simulink model "motor_model_final"  (R2020a)
settings: Solver=VariableStepAuto  StartTime=0.0  StopTime=20  RelTol=1e-3
undefined symbols (not defined in the file or in its folder): ctrl_deadZone, k_motor, Km, L, Motor, Motor_Lib, R, sigbuilder_block, X, Y, Z
libraries: fl_lib x45, nesl_utility x36, ee_lib x9, sm_lib x8, sdl_lib x3, simulink x1
(part 1 of 2)
settings Model: Creator=RAJENDRA PHUTANE  LastModifiedBy=RAJENDRA PHUTANE

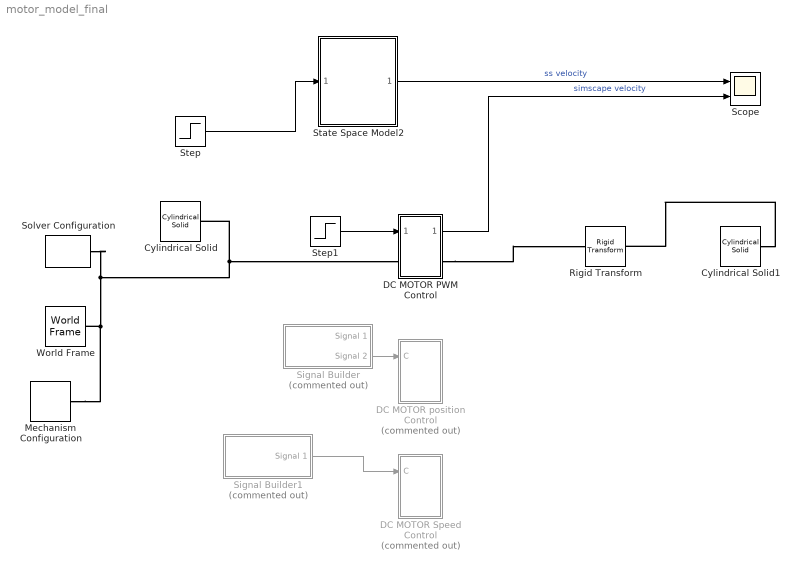
== system motor_model_final ==
  Cylindrical Solid : sm_lib/Body Elements/Cylindrical Solid  GraphicAmbientColor=[0.15 0.15 0.15 1.0]  BasedOnType=Density  CenterOfMass=[0 0 0]  CenterOfMassUnits=m  GraphicDiffuseColor=[0.5 0.5 0.5]  CylinderLength=1  CylinderLengthUnits=m  CylinderRadius=0.007  CylinderRadiusUnits=m  Density=1000  DensityUnits=kg/m^3  DoExposeReferenceFrame=on  GraphicEmissiveColor=[0.0 0.0 0.0 1.0]  ExportEntireGeometry=off  SerializedFrames=<Frames/>  MarkerShape=Sphere  MarkerSize=10  GraphicType=FromGeometry  InertiaType=CalculateFromGeometry  Mass=1  MassUnits=kg  MomentsOfInertia=[1 1 1]  MomentsOfInertiaUnits=kg*m^2  GraphicOpacity=1.0  ProductsOfInertia=[0 0 0]  ProductsOfInertiaUnits=kg*m^2  GraphicShininess=75  GraphicSpecularColor=[0.5 0.5 0.5 1.0]  GraphicVisPropType=SimpleVisualProperties
  Cylindrical Solid1 : sm_lib/Body Elements/Cylindrical Solid  GraphicAmbientColor=[0.15 0.15 0.15 1.0]  BasedOnType=Mass  CenterOfMass=[0 0 0]  CenterOfMassUnits=m  GraphicDiffuseColor=[0.5 0.5 0.5]  CylinderLength=0.01  CylinderLengthUnits=m  CylinderRadius=0.017  CylinderRadiusUnits=m  Density=1000  DensityUnits=kg/m^3  DoExposeReferenceFrame=on  GraphicEmissiveColor=[0.0 0.0 0.0 1.0]  ExportEntireGeometry=off  SerializedFrames=<Frames/>  MarkerShape=Sphere  MarkerSize=10  GraphicType=FromGeometry  InertiaType=CalculateFromGeometry  Mass=19.4  MassUnits=g  MomentsOfInertia=[1 1 1]  MomentsOfInertiaUnits=kg*m^2  GraphicOpacity=1.0  ProductsOfInertia=[0 0 0]  ProductsOfInertiaUnits=kg*m^2  GraphicShininess=75  GraphicSpecularColor=[0.5 0.5 0.5 1.0]  GraphicVisPropType=SimpleVisualProperties
  DC MOTOR PWM Control : Subsystem
  DC MOTOR Speed Control : Subsystem  Commented=on
  DC MOTOR position Control : Subsystem  Commented=on
  Mechanism Configuration : sm_lib/Utilities/Mechanism Configuration  UniformGravity=Constant  GravityVector=[0 0 -9.80665]  GravityUnits=m/s^2  LinearizationDelta=0.001
  Rigid Transform : sm_lib/Frames and Transforms/Rigid Transform  TranslationMethod=StandardAxis  TranslationStandardOffset=0.5  TranslationLengthUnit=m  TranslationStandardAxis=+Z  TranslationCartesianOffset=[0 0 0]  TranslationROffset=0  TranslationROffsetUnits=m  TranslationZOffset=0  TranslationZOffsetUnits=m  TranslationThetaOffset=0  TranslationThetaOffsetUnits=deg  RotationMethod=None  RotationAngleUnits=deg  RotationStandardAxis=+Z  RotationAngle=0.0  RotationArbitraryAxis=[0 0 1]  FollAlignAxisA=+X  BaseAlignAxisA=+Y  FollAlignAxisB=+Y  BaseAlignAxisB=+Z  RotationSequenceAxes=FollowerAxes  RotationSequence=XYX  RotationSequenceAngles=[0 0 0]  RotationSequenceAnglesUnits=deg  RotationMatrix=[1 0 0; 0 1 0; 0 0 1]
  Scope : Scope  NumInputPorts=2
  Signal Builder : Subsystem  Tag=STV Subsys  Commented=on  LoadFcn=sigbuilder_block('load');  StartFcn=sigbuilder_block('start');  StopFcn=sigbuilder_block('stop');  ClipboardFcn=sigbuilder_block('clipboard');  mask(Sigbuilder block){tuvar=[0:10]}
      mask help: Simulink:masks:SigbuilderBlock_MD
      mask init:
      | if ~strcmp(get_param(bdroot(gcbh),'SimulationStatus'),'stopped') tuvar = sigbuilder_block('maskInit'); end
      settings: CopyFcn=sigbuilder_block('copy');  DeleteFcn=sigbuilder_block('delete');  ModelCloseFcn=sigbuilder_block('modelClose');  PreSaveFcn=sigbuilder_block('preSave');  PauseFcn=sigbuilder_block('pause');  ContinueFcn=sigbuilder_block('continue');  NameChangeFcn=sigbuilder_block('namechange');  OpenFcn=sigbuilder_block('open',[437.6 199.2 550.4 400 ]);  CloseFcn=sigbuilder_block('close');
      mask Display: plot(0, 0, 100, 100,[2, 2, 32, 32, 2], [68, 8, 8, 68, 68],[32, 2], [38, 38], [32, 19, 2],[53, 60, 44], [32, 17, 17, 2],[16, 16, 31, 31]);txt = getActiveGroup(gcbh);text(2, 100, txt,'verticalAlignment', 'top');
  Signal Builder1 : Subsystem  Tag=STV Subsys  Commented=on  LoadFcn=sigbuilder_block('load');  StartFcn=sigbuilder_block('start');  StopFcn=sigbuilder_block('stop');  ClipboardFcn=sigbuilder_block('clipboard');  mask(Sigbuilder block){tuvar=[0:10]}
      mask help: Simulink:masks:SigbuilderBlock_MD
      mask init:
      | if ~strcmp(get_param(bdroot(gcbh),'SimulationStatus'),'stopped') tuvar = sigbuilder_block('maskInit'); end
      settings: CopyFcn=sigbuilder_block('copy');  DeleteFcn=sigbuilder_block('delete');  ModelCloseFcn=sigbuilder_block('modelClose');  PreSaveFcn=sigbuilder_block('preSave');  PauseFcn=sigbuilder_block('pause');  ContinueFcn=sigbuilder_block('continue');  NameChangeFcn=sigbuilder_block('namechange');  OpenFcn=sigbuilder_block('open',[437.6 199.2 550.4 400 ]);  CloseFcn=sigbuilder_block('close');
      mask Display: plot(0, 0, 100, 100,[2, 2, 32, 32, 2], [68, 8, 8, 68, 68],[32, 2], [38, 38], [32, 19, 2],[53, 60, 44], [32, 17, 17, 2],[16, 16, 31, 31]);txt = getActiveGroup(gcbh);text(2, 100, txt,'verticalAlignment', 'top');
  Solver Configuration : nesl_utility/Solver Configuration  PhysicalDomain=network_engine_domain  SubClassName=solver  LeftPortType=input  RightPortType=generic  Tones=[]  Harmonics=[]  SimulateNoise=off  Profile=off  UseLocalSampling=off  EnableSwitchedLinearOptims=on  FrequencyDomain=off  UseCCode=off  RelTol=0.001  AbsTol=1e-06  MinStep=1e-09  ToWorkspace=off  RevertToSquareIcSolve=off  NumHomotopyIterations=100  PhasorMode=off  PhasorModeNumHarmonics=1  DoDC=off  ResidualTolerance=1e-09  UseLocalSolver=off  LocalSolverChoice=NE_BACKWARD_EULER_ADVANCER  LocalSolverSampleTime=0.001  DoFixedCost=off  MaxNonlinIter=3  MaxModeIter=2  LinearAlgebra=auto  EquationFormulation=NE_TIME_EF  DelaysMemoryBudget=1024  AutomaticFiltering=on  FilteringTimeConstant=0.001  PartitionStorageMethod=AS_NEEDED  PartitionMemoryBudget=1024  PartitionMethod=ROBUST
  State Space Model2 : Subsystem  AncestorBlock=DCMotorLibrary/State Space Model  mask(DC Motor){K=Km, R=R, L=L, b=0.0005625, J=0.0001}
      mask prompts: K "Torque Constant:"; R "Armature Resistance:"; L "Armature Inductance:"; b "Damping Coefficient:"; J "Rotor Inertia:"
      mask help:
      | This block simulates a basic brushed DC Motor with voltage input and rotor
      | angle in degrees as the output.
      mask Display: image(imread('dcmotor.jpg'))
  Step : Step  Time=5  Before=-12  After=12  SampleTime=0
  Step1 : Step  Time=5  Before=-255  After=255  SampleTime=0
  World Frame : sm_lib/Frames and Transforms/World Frame
  wires:
  Step1/1 -> DC MOTOR PWM Control/1(PWM)
  Signal Builder/2(Signal 2) -> DC MOTOR position Control/1(C)
  Signal Builder1/1(Signal 1) -> DC MOTOR Speed Control/1(C)
  DC MOTOR PWM Control/1(Outport) -> Scope/2  "simscape velocity"
  Step/1 -> State Space Model2/1(Voltage)
  State Space Model2/1(Velocity) -> Scope/1  "ss velocity"
  connections:
  Cylindrical Solid1/RConn1 -- Rigid Transform/RConn1
  Mechanism Configuration/RConn1 -- Solver Configuration/RConn1 -- DC MOTOR PWM Control/LConn1 -- Cylindrical Solid/RConn1 -- World Frame/RConn1
  DC MOTOR PWM Control/RConn1 -- Rigid Transform/LConn1

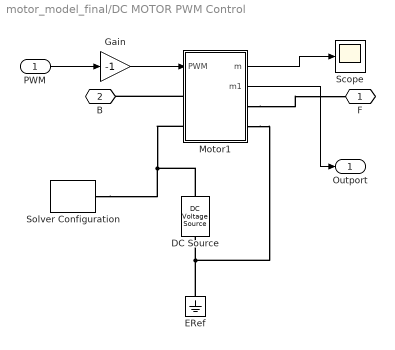
== system motor_model_final/DC MOTOR PWM Control ==
  PWM : Inport
  DC Source : fl_lib/Electrical/Electrical Sources/DC Voltage Source  v0=12 V
  ERef : fl_lib/Electrical/Electrical Elements/Electrical Reference
  Gain : Gain  Gain=-1
  Motor1 : Subsystem  VariantControl=Motor
      mask Display: image('youBot_Arm_Actuation_Motor_Motor_IMAGE.jpg');
  Scope : Scope
  Solver Configuration : nesl_utility/Solver Configuration  PhysicalDomain=network_engine_domain  SubClassName=solver  LeftPortType=input  RightPortType=generic  Tones=[]  Harmonics=[]  SimulateNoise=off  Profile=off  UseLocalSampling=off  EnableSwitchedLinearOptims=on  FrequencyDomain=off  UseCCode=off  RelTol=0.001  AbsTol=1e-06  MinStep=1e-09  ToWorkspace=off  RevertToSquareIcSolve=off  NumHomotopyIterations=100  PhasorMode=off  PhasorModeNumHarmonics=1  DoDC=off  ResidualTolerance=1e-09  UseLocalSolver=off  LocalSolverChoice=NE_BACKWARD_EULER_ADVANCER  LocalSolverSampleTime=0.001  DoFixedCost=off  MaxNonlinIter=3  MaxModeIter=2  LinearAlgebra=auto  EquationFormulation=NE_TIME_EF  DelaysMemoryBudget=1024  AutomaticFiltering=on  FilteringTimeConstant=0.001  PartitionStorageMethod=AS_NEEDED  PartitionMemoryBudget=1024  PartitionMethod=ROBUST
  F : PMIOPort  Side=Right
  B : PMIOPort  Port=2  Side=Left
  Outport : Outport
  wires:
  PWM/1 -> Gain/1
  Motor1/1(m) -> Scope/1
  Gain/1 -> Motor1/1(PWM)
  Motor1/2(m1) -> Outport/1
  connections:
  Motor1/RConn1 -- F/RConn1
  Motor1/LConn1 -- B/RConn1
  Solver Configuration/RConn1 -- Motor1/LConn2 -- DC Source/LConn1
  ERef/LConn1 -- Motor1/RConn2 -- DC Source/RConn1

== system motor_model_final/DC MOTOR Speed Control ==
  C : Inport
  DC Source : fl_lib/Electrical/Electrical Sources/DC Voltage Source  v0=12 V
  ERef : fl_lib/Electrical/Electrical Elements/Electrical Reference
  Motor1 : Subsystem  VariantControl=Motor
      mask Display: image('youBot_Arm_Actuation_Motor_Motor_IMAGE.jpg');
  Solver Configuration : nesl_utility/Solver Configuration  PhysicalDomain=network_engine_domain  SubClassName=solver  LeftPortType=input  RightPortType=generic  Tones=[]  Harmonics=[]  SimulateNoise=off  Profile=off  UseLocalSampling=off  EnableSwitchedLinearOptims=on  FrequencyDomain=off  UseCCode=off  RelTol=0.001  AbsTol=1e-06  MinStep=1e-09  ToWorkspace=off  RevertToSquareIcSolve=off  NumHomotopyIterations=100  PhasorMode=off  PhasorModeNumHarmonics=1  DoDC=off  ResidualTolerance=1e-09  UseLocalSolver=off  LocalSolverChoice=NE_BACKWARD_EULER_ADVANCER  LocalSolverSampleTime=0.001  DoFixedCost=off  MaxNonlinIter=3  MaxModeIter=2  LinearAlgebra=auto  EquationFormulation=NE_TIME_EF  DelaysMemoryBudget=1024  AutomaticFiltering=on  FilteringTimeConstant=0.001  PartitionStorageMethod=AS_NEEDED  PartitionMemoryBudget=1024  PartitionMethod=ROBUST
  Terminator : Terminator
  F : PMIOPort  Side=Right
  B : PMIOPort  Port=2  Side=Left
  wires:
  C/1 -> Motor1/1(C)
  Motor1/1(m) -> Terminator/1
  connections:
  Motor1/RConn1 -- F/RConn1
  Motor1/LConn1 -- B/RConn1
  Solver Configuration/RConn1 -- Motor1/LConn2 -- DC Source/LConn1
  ERef/LConn1 -- Motor1/RConn2 -- DC Source/RConn1

== system motor_model_final/DC MOTOR position Control ==
  C : Inport
  DC Source : fl_lib/Electrical/Electrical Sources/DC Voltage Source  v0=12 V
  ERef : fl_lib/Electrical/Electrical Elements/Electrical Reference
  Motor1 : Subsystem  VariantControl=Motor
      mask Display: image('youBot_Arm_Actuation_Motor_Motor_IMAGE.jpg');
  Solver Configuration : nesl_utility/Solver Configuration  PhysicalDomain=network_engine_domain  SubClassName=solver  LeftPortType=input  RightPortType=generic  Tones=[]  Harmonics=[]  SimulateNoise=off  Profile=off  UseLocalSampling=off  EnableSwitchedLinearOptims=on  FrequencyDomain=off  UseCCode=off  RelTol=0.001  AbsTol=1e-06  MinStep=1e-09  ToWorkspace=off  RevertToSquareIcSolve=off  NumHomotopyIterations=100  PhasorMode=off  PhasorModeNumHarmonics=1  DoDC=off  ResidualTolerance=1e-09  UseLocalSolver=off  LocalSolverChoice=NE_BACKWARD_EULER_ADVANCER  LocalSolverSampleTime=0.001  DoFixedCost=off  MaxNonlinIter=3  MaxModeIter=2  LinearAlgebra=auto  EquationFormulation=NE_TIME_EF  DelaysMemoryBudget=1024  AutomaticFiltering=on  FilteringTimeConstant=0.001  PartitionStorageMethod=AS_NEEDED  PartitionMemoryBudget=1024  PartitionMethod=ROBUST
  Terminator : Terminator
  F : PMIOPort  Side=Right
  B : PMIOPort  Port=2  Side=Left
  wires:
  Motor1/1(m) -> Terminator/1
  C/1 -> Motor1/1(C)
  connections:
  DC Source/RConn1 -- Motor1/RConn2 -- ERef/LConn1
  DC Source/LConn1 -- Motor1/LConn2 -- Solver Configuration/RConn1
  Motor1/LConn1 -- B/RConn1
  Motor1/RConn1 -- F/RConn1

== system motor_model_final/Signal Builder ==
  Demux : Demux  Tag=STV Demux  Outputs=2
      settings: DisplayOption=none
  FromWs : FromWorkspace  Tag=STV FromWs  VariableName=tuvar
      SigBuilderData=|
      | common.afterFinalStr = 'Extrapolate'
      | common.sampleTime = 0
      | dataSet.timeRange = [0 10]
      | dataSet.name = 'Group 1'
      | sbobj.Groups.Name = 'Group 1'
      | sbobj.Groups.Signals(1).Name = 'Signal 1'
      | sbobj.Groups.Signals(1).XData = [0 4 4 6 6 10]
      | sbobj.Groups.Signals(1).YData = [0 0 1 1 0 0]
      | sbobj.Groups.Signals(2).Name = 'Signal 2'
      | sbobj.Groups.Signals(2).XData = [0 2 3 4 5 6 10]
      | sbobj.Groups.Signals(2).YData = [0 180 180 90 90 -90 -90]
  Signal 1 : Outport  Tag=STV Outport
  Signal 2 : Outport  Tag=STV Outport  Port=2
  wires:
  Demux/1 -> Signal 1/1
  FromWs/1 -> Demux/1
  Demux/2 -> Signal 2/1

== system motor_model_final/Signal Builder1 ==
  Demux : Demux  Tag=STV Demux  Outputs=1
      settings: DisplayOption=none
  FromWs : FromWorkspace  Tag=STV FromWs  VariableName=tuvar
      SigBuilderData=|
      | common.afterFinalStr = 'Extrapolate'
      | common.sampleTime = 0
      | dataSet.timeRange = [0 20]
      | dataSet.name = 'Group 1'
      | sbobj.Groups.Name = 'Group 1'
      | sbobj.Groups.Signals.Name = 'Signal 1'
      | sbobj.Groups.Signals.XData = [0 1 1 3.98 3.98 6 6 9 9 14 14 20]
      | sbobj.Groups.Signals.YData = [0 0 0.6 0.6 0 0 -0.5 -0.5 0 0.5 -0.685 -0.685]
      | sbobj.Groups.TimeRange = [0 20]
  Signal 1 : Outport  Tag=STV Outport
  wires:
  Demux/1 -> Signal 1/1
  FromWs/1 -> Demux/1

== system motor_model_final/State Space Model2 ==
  Voltage : Inport
  State-Space : StateSpace  A=[-b/J K/J; -K/L -R/L]  B=[0; 1/L]  C=[1 0]  D=[0]  InitialCondition=0
  Velocity : Outport
  wires:
  Voltage/1 -> State-Space/1
  State-Space/1 -> Velocity/1

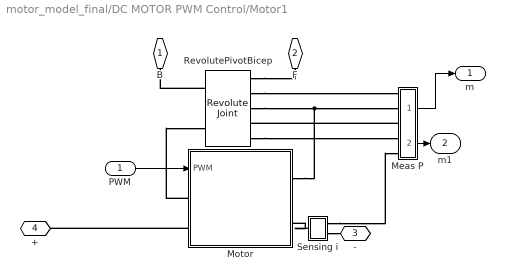
== system motor_model_final/DC MOTOR PWM Control/Motor1 ==
  PWM : Inport
  Meas P : Subsystem  Tag=CustomStyle
      mask Display: disp('m')
  Motor : Subsystem  AncestorBlock=Motor_Lib/Motor  VariantControl=Motor
  RevolutePivotBicep : sm_lib/Joints/Revolute Joint  JointMode=Normal  SenseConstraintForce=on  SenseConstraintForceX=off  SenseConstraintForceY=off  SenseConstraintForceZ=off  SenseConstraintTorque=off  SenseConstraintTorqueX=off  SenseConstraintTorqueY=off  SenseConstraintTorqueZ=off  SenseTotalForce=off  SenseTotalForceX=off  SenseTotalForceY=off  SenseTotalForceZ=off  SenseTotalTorque=off  SenseTotalTorqueX=off  SenseTotalTorqueY=off  SenseTotalTorqueZ=off  CompositeWrenchDir=FollowerOnBase  CompositeWrenchFrame=BaseFrame  EquilibriumPosition=0  EquilibriumPositionUnits=rad  SpringStiffness=0  SpringStiffnessUnits=N*m/rad  DampingCoefficient=0  DampingCoefficientUnits=N*m/(rad/s)  TorqueActuationMode=InputTorque  MotionActuationMode=ComputedMotion  SensePosition=on  SenseVelocity=on  SenseAcceleration=off  SenseTorqueForce=on  SenseLowerLimitTorqueForce=off  SenseUpperLimitTorqueForce=off  LowerLimitSpecify=off  LowerLimitBound=-90  LowerLimitBoundUnits=deg  LowerLimitStiffness=1e4  LowerLimitStiffnessUnits=N*m/deg  LowerLimitDamping=10  LowerLimitDampingUnits=N*m/(deg/s)  LowerLimitTransitionRegionWidth=0.1  LowerLimitTransitionRegionWidthUnits=deg  UpperLimitSpecify=off  UpperLimitBound=90  UpperLimitBoundUnits=deg  UpperLimitStiffness=1e4  UpperLimitStiffnessUnits=N*m/deg  UpperLimitDamping=10  UpperLimitDampingUnits=N*m/(deg/s)  UpperLimitTransitionRegionWidth=0.1  UpperLimitTransitionRegionWidthUnits=deg  PositionTargetSpecify=on  PositionTargetPriority=Low  PositionTargetValue=0  PositionTargetValueUnits=deg  VelocityTargetSpecify=off  VelocityTargetPriority=High  VelocityTargetValue=0  VelocityTargetValueUnits=deg/s
  Sensing i : Subsystem
      mask Display: disp('i')
  B : PMIOPort  Side=Left
  F : PMIOPort  Port=2  Side=Right
  - : PMIOPort  Port=3  Side=Right
  + : PMIOPort  Port=4  Side=Left
  m : Outport  VectorParamsAs1DForOutWhenUnconnected=off
  m1 : Outport  Port=2  VectorParamsAs1DForOutWhenUnconnected=off
  wires:
  PWM/1 -> Motor/1(PWM)
  Meas P/1(P) -> m/1
  Meas P/2(P1) -> m1/1
  connections:
  RevolutePivotBicep/RConn5 -- Meas P/LConn4
  Sensing i/RConn1 -- Meas P/LConn5
  Sensing i/RConn2 -- -/RConn1
  Motor/LConn2 -- +/RConn1
  Sensing i/LConn1 -- Motor/RConn2
  RevolutePivotBicep/LConn1 -- B/RConn1
  RevolutePivotBicep/RConn1 -- F/RConn1
  Motor/LConn1 -- RevolutePivotBicep/LConn2
  Motor/RConn1 -- RevolutePivotBicep/RConn3 -- Meas P/LConn2
  Meas P/LConn3 -- RevolutePivotBicep/RConn4
  RevolutePivotBicep/RConn2 -- Meas P/LConn1

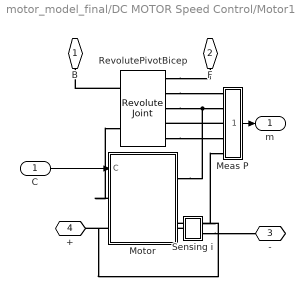
== system motor_model_final/DC MOTOR Speed Control/Motor1 ==
  C : Inport
  Meas P : Subsystem  Tag=CustomStyle
      mask Display: disp('m')
  Motor : Subsystem  AncestorBlock=Motor_Lib/Motor  VariantControl=Motor
  RevolutePivotBicep : sm_lib/Joints/Revolute Joint  JointMode=Normal  SenseConstraintForce=on  SenseConstraintForceX=off  SenseConstraintForceY=off  SenseConstraintForceZ=off  SenseConstraintTorque=off  SenseConstraintTorqueX=off  SenseConstraintTorqueY=off  SenseConstraintTorqueZ=off  SenseTotalForce=off  SenseTotalForceX=off  SenseTotalForceY=off  SenseTotalForceZ=off  SenseTotalTorque=off  SenseTotalTorqueX=off  SenseTotalTorqueY=off  SenseTotalTorqueZ=off  CompositeWrenchDir=FollowerOnBase  CompositeWrenchFrame=BaseFrame  EquilibriumPosition=0  EquilibriumPositionUnits=rad  SpringStiffness=0  SpringStiffnessUnits=N*m/rad  DampingCoefficient=0  DampingCoefficientUnits=N*m/(rad/s)  TorqueActuationMode=InputTorque  MotionActuationMode=ComputedMotion  SensePosition=on  SenseVelocity=on  SenseAcceleration=off  SenseTorqueForce=on  SenseLowerLimitTorqueForce=off  SenseUpperLimitTorqueForce=off  LowerLimitSpecify=off  LowerLimitBound=-90  LowerLimitBoundUnits=deg  LowerLimitStiffness=1e4  LowerLimitStiffnessUnits=N*m/deg  LowerLimitDamping=10  LowerLimitDampingUnits=N*m/(deg/s)  LowerLimitTransitionRegionWidth=0.1  LowerLimitTransitionRegionWidthUnits=deg  UpperLimitSpecify=off  UpperLimitBound=90  UpperLimitBoundUnits=deg  UpperLimitStiffness=1e4  UpperLimitStiffnessUnits=N*m/deg  UpperLimitDamping=10  UpperLimitDampingUnits=N*m/(deg/s)  UpperLimitTransitionRegionWidth=0.1  UpperLimitTransitionRegionWidthUnits=deg  PositionTargetSpecify=on  PositionTargetPriority=Low  PositionTargetValue=0  PositionTargetValueUnits=deg  VelocityTargetSpecify=off  VelocityTargetPriority=High  VelocityTargetValue=0  VelocityTargetValueUnits=deg/s
  Sensing i : Subsystem
      mask Display: disp('i')
  B : PMIOPort  Side=Left
  F : PMIOPort  Port=2  Side=Right
  - : PMIOPort  Port=3  Side=Right
  + : PMIOPort  Port=4  Side=Left
  m : Outport  VectorParamsAs1DForOutWhenUnconnected=off
  wires:
  C/1 -> Motor/1(C)
  Meas P/1(P) -> m/1
  connections:
  RevolutePivotBicep/RConn5 -- Meas P/LConn4
  Sensing i/RConn1 -- Meas P/LConn5
  Sensing i/RConn2 -- -/RConn1
  Motor/LConn2 -- +/RConn1
  Sensing i/LConn1 -- Motor/RConn2
  RevolutePivotBicep/LConn1 -- B/RConn1
  RevolutePivotBicep/RConn1 -- F/RConn1
  Motor/LConn1 -- RevolutePivotBicep/LConn2
  Motor/RConn1 -- Meas P/LConn2 -- RevolutePivotBicep/RConn3
  Meas P/LConn3 -- RevolutePivotBicep/RConn4
  RevolutePivotBicep/RConn2 -- Meas P/LConn1

== system motor_model_final/DC MOTOR position Control/Motor1 ==
  C : Inport
  Meas P : Subsystem  Tag=CustomStyle
      mask Display: disp('m')
  Motor : Subsystem  AncestorBlock=Motor_Lib/Motor  VariantControl=Motor
  RevolutePivotBicep : sm_lib/Joints/Revolute Joint  JointMode=Normal  SenseConstraintForce=on  SenseConstraintForceX=off  SenseConstraintForceY=off  SenseConstraintForceZ=off  SenseConstraintTorque=off  SenseConstraintTorqueX=off  SenseConstraintTorqueY=off  SenseConstraintTorqueZ=off  SenseTotalForce=off  SenseTotalForceX=off  SenseTotalForceY=off  SenseTotalForceZ=off  SenseTotalTorque=off  SenseTotalTorqueX=off  SenseTotalTorqueY=off  SenseTotalTorqueZ=off  CompositeWrenchDir=FollowerOnBase  CompositeWrenchFrame=BaseFrame  EquilibriumPosition=0  EquilibriumPositionUnits=rad  SpringStiffness=0  SpringStiffnessUnits=N*m/rad  DampingCoefficient=0  DampingCoefficientUnits=N*m/(rad/s)  TorqueActuationMode=InputTorque  MotionActuationMode=ComputedMotion  SensePosition=on  SenseVelocity=on  SenseAcceleration=off  SenseTorqueForce=on  SenseLowerLimitTorqueForce=off  SenseUpperLimitTorqueForce=off  LowerLimitSpecify=off  LowerLimitBound=-90  LowerLimitBoundUnits=deg  LowerLimitStiffness=1e4  LowerLimitStiffnessUnits=N*m/deg  LowerLimitDamping=10  LowerLimitDampingUnits=N*m/(deg/s)  LowerLimitTransitionRegionWidth=0.1  LowerLimitTransitionRegionWidthUnits=deg  UpperLimitSpecify=off  UpperLimitBound=90  UpperLimitBoundUnits=deg  UpperLimitStiffness=1e4  UpperLimitStiffnessUnits=N*m/deg  UpperLimitDamping=10  UpperLimitDampingUnits=N*m/(deg/s)  UpperLimitTransitionRegionWidth=0.1  UpperLimitTransitionRegionWidthUnits=deg  PositionTargetSpecify=on  PositionTargetPriority=Low  PositionTargetValue=0  PositionTargetValueUnits=deg  VelocityTargetSpecify=off  VelocityTargetPriority=High  VelocityTargetValue=0  VelocityTargetValueUnits=deg/s
  Sensing i : Subsystem
      mask Display: disp('i')
  B : PMIOPort  Side=Left
  F : PMIOPort  Port=2  Side=Right
  - : PMIOPort  Port=3  Side=Right
  + : PMIOPort  Port=4  Side=Left
  m : Outport  VectorParamsAs1DForOutWhenUnconnected=off
  wires:
  Meas P/1(P) -> m/1
  C/1 -> Motor/1(C)
  connections:
  RevolutePivotBicep/RConn2 -- Motor/RConn1 -- Meas P/LConn1
  Meas P/LConn3 -- RevolutePivotBicep/RConn4
  RevolutePivotBicep/RConn3 -- Meas P/LConn2 -- Motor/RConn2
  Motor/LConn1 -- RevolutePivotBicep/LConn2
  RevolutePivotBicep/RConn1 -- F/RConn1
  RevolutePivotBicep/LConn1 -- B/RConn1
  Sensing i/LConn1 -- Motor/RConn3
  Motor/LConn2 -- +/RConn1
  Sensing i/RConn2 -- -/RConn1
  Sensing i/RConn1 -- Meas P/LConn5
  RevolutePivotBicep/RConn5 -- Meas P/LConn4

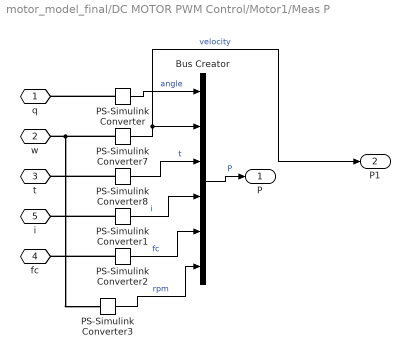
== system motor_model_final/DC MOTOR PWM Control/Motor1/Meas P ==
  Bus Creator : BusCreator  Inputs=6
  PS-Simulink Converter : nesl_utility/PS-Simulink Converter  PhysicalDomain=network_engine_domain  SubClassName=ps_output  LeftPortType=input  RightPortType=output  PseudoPeriodic=off  Frequencies=[]  Unit=rad  AffineConversion=off
  PS-Simulink Converter1 : nesl_utility/PS-Simulink Converter  PhysicalDomain=network_engine_domain  SubClassName=ps_output  LeftPortType=input  RightPortType=output  PseudoPeriodic=off  Frequencies=[]  Unit=A  AffineConversion=off
  PS-Simulink Converter2 : nesl_utility/PS-Simulink Converter  PhysicalDomain=network_engine_domain  SubClassName=ps_output  LeftPortType=input  RightPortType=output  PseudoPeriodic=off  Frequencies=[]  Unit=1  AffineConversion=off
  PS-Simulink Converter3 : nesl_utility/PS-Simulink Converter  PhysicalDomain=network_engine_domain  SubClassName=ps_output  LeftPortType=input  RightPortType=output  PseudoPeriodic=off  Frequencies=[]  Unit=rpm  AffineConversion=off
  PS-Simulink Converter7 : nesl_utility/PS-Simulink Converter  PhysicalDomain=network_engine_domain  SubClassName=ps_output  LeftPortType=input  RightPortType=output  PseudoPeriodic=off  Frequencies=[]  Unit=rad/s  AffineConversion=off
  PS-Simulink Converter8 : nesl_utility/PS-Simulink Converter  PhysicalDomain=network_engine_domain  SubClassName=ps_output  LeftPortType=input  RightPortType=output  PseudoPeriodic=off  Frequencies=[]  Unit=N*m  AffineConversion=off
  q : PMIOPort  Side=Left
  w : PMIOPort  Port=2  Side=Left
  t : PMIOPort  Port=3  Side=Left
  fc : PMIOPort  Port=4  Side=Left
  i : PMIOPort  Port=5  Side=Left
  P : Outport  VectorParamsAs1DForOutWhenUnconnected=off
  P1 : Outport  Port=2  VectorParamsAs1DForOutWhenUnconnected=off
  wires:
  PS-Simulink Converter3/1 -> Bus Creator/6  "rpm"
  PS-Simulink Converter2/1 -> Bus Creator/5  "fc"
  PS-Simulink Converter1/1 -> Bus Creator/4  "i"
  PS-Simulink Converter/1 -> Bus Creator/1  "angle"
  PS-Simulink Converter7/1 -> P1/1, Bus Creator/2  "velocity"
  PS-Simulink Converter8/1 -> Bus Creator/3  "t"
  Bus Creator/1 -> P/1  "P"
  connections:
  w/RConn1 -- PS-Simulink Converter3/LConn1 -- PS-Simulink Converter7/LConn1
  PS-Simulink Converter2/LConn1 -- fc/RConn1
  PS-Simulink Converter1/LConn1 -- i/RConn1
  PS-Simulink Converter/LConn1 -- q/RConn1
  PS-Simulink Converter8/LConn1 -- t/RConn1

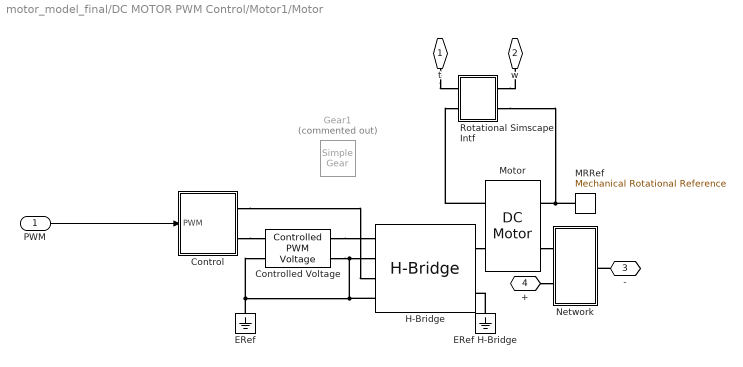
== system motor_model_final/DC MOTOR PWM Control/Motor1/Motor ==
  PWM : Inport
  Control : Subsystem
  Controlled Voltage : ee_lib/Integrated Circuits/Controlled PWM Voltage  F=1000 Hz  TD=0 s  pulse_width_offset=0 s  pulse_min=0 s  Vmin=0 V  Vmax=5 V  Vm=5 V  pwm_or_av=2  event_type=1  sample_time=1e-6 s  u_min=0  u_max=1
  ERef : fl_lib/Electrical/Electrical Elements/Electrical Reference
  ERef H-Bridge : fl_lib/Electrical/Electrical Elements/Electrical Reference
  Gear1 : sdl_lib/Gears/Simple Gear  Commented=on  ratio=1  rotation_direction=1  friction_model=sdl.enum.gear_efficiencies_load.off  T_noload=0.1 N*m  T_nom=5 N*m  efficiency_nom=0.8  efficiency=0.8  mu_visc=[ 0 0 ] N*m/(rad/s)  w_thr=0.01 rad/s  pwr_thr=0.001 W  enable_faults=simscape.enum.onoff.off  efficiency_fault=0.05  external_fault=simscape.enum.onoff.off  temporal_fault=simscape.enum.onoff.off  fault_time=5 s  fault_angles=pi / 12 rad  report_fault=1  temperature_TLU=[ 280 300 320 ] K  load_TLU=[ 1 5 10 ] N*m  efficiency_TLU=[ 0.95 0.9 0.85 ]  efficiency_TLU2=[ 0.85 0.8 0.75; 0.95 0.9 0.85; 0.85 0.8 0.7 ]  thermal_mass=50 J/K  T_init=300 K
  H-Bridge : ee_lib/Semiconductors & Converters/Converters/H-Bridge  supply_ports=ee.enum.supply_ports.hidesupply  Venable=2.5 V  Vmax=5.0 V  Vreverse=2.5 V  Vbrake=2.5 V  Vm=12 V  pwm_or_av=ee.enum.pwm_or_av.averaged  regenerative_braking_mode=ee.enum.converters.regenerative_braking_mode.always_enabled  discontinuous=ee.enum.current_profile.continuous  freewheeling_mode=ee.enum.converters.freewheeling_mode.one_switch_one_diode  Ron=0.1 Ohm  Don=0.05 Ohm  Goff=1e-6 S  Rload=10 Ohm  Lload=1e-5 H  F=10 kHz  thermal_mass=100 J/K  initial_temperature=298.15 K  Ron2=0.1 Ohm  Don2=0.05 Ohm  Tmeas=298.15 K  Tmeas2=398.15 K
  MRRef : fl_lib/Mechanical/Rotational Elements/Mechanical Rotational Reference
  Motor : ee_lib/Electromechanical/Brushed Motors/DC Motor  field_option=ee.enum.field_option.pm  Rf=100 Ohm  Lf=1 H  Laf=0.15 H  If0=0 A  parameterization=ee.enum.dcparam_option.torque_speed  Ra=R Ohm  La=L H  emf_or_torque=ee.enum.emf_or_torque.ki  Kv=YBT_Par.Pivot.Motor.K V/rpm  Ki=Km N*m/A  T_stall=0.0637 N*m  w_max=600 rpm  w_rated=1.5e+4 rpm  P_rated=0.08 W  V_rated=12 V  J=0.0001 kg*m^2  lam_param=ee.enum.lam_param.current  lam=0.00058 N*m/(rad/s)  i_noload=0.06 A  V_i_noload=12 V  speed0=0 rpm  alpha=3.93e-3 1/K  Tmeas=25 degC  thermal_mass=100 J/K  initial_temperature=25 degC
  Network : Subsystem
  Rotational Simscape Intf : Subsystem
  t : PMIOPort  Side=Left
  w : PMIOPort  Port=2  Side=Right
  - : PMIOPort  Port=3  Side=Right
  + : PMIOPort  Port=4  Side=Left
  wires:
  PWM/1 -> Control/1(PWM)
  connections:
  Rotational Simscape Intf/RConn1 -- w/RConn1
  +/RConn1 -- Network/LConn2
  -/RConn1 -- Network/RConn1
  Motor/RConn1 -- Network/LConn1
  ERef H-Bridge/LConn1 -- H-Bridge/RConn2
  Control/RConn1 -- H-Bridge/LConn3
  Control/RConn2 -- Controlled Voltage/LConn1
  H-Bridge/RConn1 -- Motor/LConn1
  H-Bridge/LConn4 -- Controlled Voltage/LConn2 -- ERef/LConn1 -- H-Bridge/LConn2 -- Controlled Voltage/RConn2
  Controlled Voltage/RConn1 -- H-Bridge/LConn1
  t/RConn1 -- Rotational Simscape Intf/LConn1
  Rotational Simscape Intf/RConn2 -- MRRef/LConn1 -- Motor/RConn2
  Motor/LConn2 -- Rotational Simscape Intf/LConn2

== system motor_model_final/DC MOTOR PWM Control/Motor1/Sensing i ==
  Current Sensor : fl_lib/Electrical/Electrical Sensors/Current Sensor
  i : PMIOPort  Side=Right
  + : PMIOPort  Port=2  Side=Left
  - : PMIOPort  Port=3  Side=Right
  connections:
  Current Sensor/LConn1 -- +/RConn1
  Current Sensor/RConn2 -- -/RConn1
  Current Sensor/RConn1 -- i/RConn1

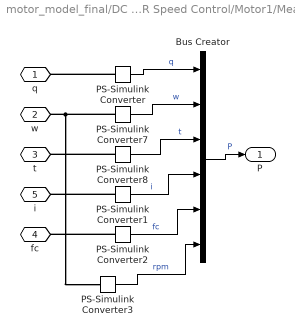
== system motor_model_final/DC MOTOR Speed Control/Motor1/Meas P ==
  Bus Creator : BusCreator  Inputs=6
  PS-Simulink Converter : nesl_utility/PS-Simulink Converter  PhysicalDomain=network_engine_domain  SubClassName=ps_output  LeftPortType=input  RightPortType=output  PseudoPeriodic=off  Frequencies=[]  Unit=rad  AffineConversion=off
  PS-Simulink Converter1 : nesl_utility/PS-Simulink Converter  PhysicalDomain=network_engine_domain  SubClassName=ps_output  LeftPortType=input  RightPortType=output  PseudoPeriodic=off  Frequencies=[]  Unit=A  AffineConversion=off
  PS-Simulink Converter2 : nesl_utility/PS-Simulink Converter  PhysicalDomain=network_engine_domain  SubClassName=ps_output  LeftPortType=input  RightPortType=output  PseudoPeriodic=off  Frequencies=[]  Unit=1  AffineConversion=off
  PS-Simulink Converter3 : nesl_utility/PS-Simulink Converter  PhysicalDomain=network_engine_domain  SubClassName=ps_output  LeftPortType=input  RightPortType=output  PseudoPeriodic=off  Frequencies=[]  Unit=rpm  AffineConversion=off
  PS-Simulink Converter7 : nesl_utility/PS-Simulink Converter  PhysicalDomain=network_engine_domain  SubClassName=ps_output  LeftPortType=input  RightPortType=output  PseudoPeriodic=off  Frequencies=[]  Unit=rad/s  AffineConversion=off
  PS-Simulink Converter8 : nesl_utility/PS-Simulink Converter  PhysicalDomain=network_engine_domain  SubClassName=ps_output  LeftPortType=input  RightPortType=output  PseudoPeriodic=off  Frequencies=[]  Unit=N*m  AffineConversion=off
  q : PMIOPort  Side=Left
  w : PMIOPort  Port=2  Side=Left
  t : PMIOPort  Port=3  Side=Left
  fc : PMIOPort  Port=4  Side=Left
  i : PMIOPort  Port=5  Side=Left
  P : Outport  VectorParamsAs1DForOutWhenUnconnected=off
  wires:
  PS-Simulink Converter3/1 -> Bus Creator/6  "rpm"
  PS-Simulink Converter2/1 -> Bus Creator/5  "fc"
  PS-Simulink Converter1/1 -> Bus Creator/4  "i"
  PS-Simulink Converter/1 -> Bus Creator/1  "q"
  PS-Simulink Converter7/1 -> Bus Creator/2  "w"
  PS-Simulink Converter8/1 -> Bus Creator/3  "t"
  Bus Creator/1 -> P/1  "P"
  connections:
  w/RConn1 -- PS-Simulink Converter3/LConn1 -- PS-Simulink Converter7/LConn1
  PS-Simulink Converter2/LConn1 -- fc/RConn1
  PS-Simulink Converter1/LConn1 -- i/RConn1
  PS-Simulink Converter/LConn1 -- q/RConn1
  PS-Simulink Converter8/LConn1 -- t/RConn1

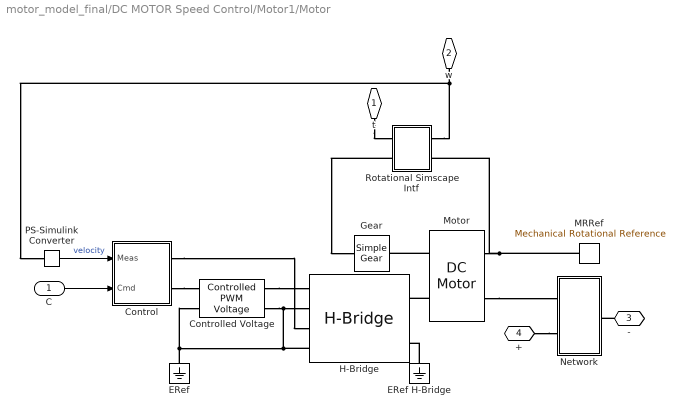
== system motor_model_final/DC MOTOR Speed Control/Motor1/Motor ==
  C : Inport
  Control : Subsystem
  Controlled Voltage : ee_lib/Integrated Circuits/Controlled PWM Voltage  F=1000 Hz  TD=0 s  pulse_width_offset=0 s  pulse_min=0 s  Vmin=0 V  Vmax=5 V  Vm=5 V  pwm_or_av=2  event_type=1  sample_time=1e-6 s  u_min=0  u_max=1
  ERef : fl_lib/Electrical/Electrical Elements/Electrical Reference
  ERef H-Bridge : fl_lib/Electrical/Electrical Elements/Electrical Reference
  Gear : sdl_lib/Gears/Simple Gear  ratio=1  rotation_direction=1  friction_model=sdl.enum.gear_efficiencies_load.off  T_noload=0.1 N*m  T_nom=5 N*m  efficiency_nom=0.8  efficiency=0.8  mu_visc=[ 0 0 ] N*m/(rad/s)  w_thr=0.01 rad/s  pwr_thr=0.001 W  enable_faults=simscape.enum.onoff.off  efficiency_fault=0.05  external_fault=simscape.enum.onoff.off  temporal_fault=simscape.enum.onoff.off  fault_time=5 s  fault_angles=pi / 12 rad  report_fault=1  temperature_TLU=[ 280 300 320 ] K  load_TLU=[ 1 5 10 ] N*m  efficiency_TLU=[ 0.95 0.9 0.85 ]  efficiency_TLU2=[ 0.85 0.8 0.75; 0.95 0.9 0.85; 0.85 0.8 0.7 ]  thermal_mass=50 J/K  T_init=300 K
  H-Bridge : ee_lib/Semiconductors & Converters/Converters/H-Bridge  supply_ports=ee.enum.supply_ports.hidesupply  Venable=2.5 V  Vmax=5.0 V  Vreverse=2.5 V  Vbrake=2.5 V  Vm=12 V  pwm_or_av=ee.enum.pwm_or_av.averaged  regenerative_braking_mode=ee.enum.converters.regenerative_braking_mode.always_enabled  discontinuous=ee.enum.current_profile.continuous  freewheeling_mode=ee.enum.converters.freewheeling_mode.one_switch_one_diode  Ron=0.1 Ohm  Don=0.05 Ohm  Goff=1e-6 S  Rload=10 Ohm  Lload=1e-5 H  F=10 kHz  thermal_mass=100 J/K  initial_temperature=298.15 K  Ron2=0.1 Ohm  Don2=0.05 Ohm  Tmeas=298.15 K  Tmeas2=398.15 K
  MRRef : fl_lib/Mechanical/Rotational Elements/Mechanical Rotational Reference
  Motor : ee_lib/Electromechanical/Brushed Motors/DC Motor  field_option=ee.enum.field_option.pm  Rf=100 Ohm  Lf=1 H  Laf=0.15 H  If0=0 A  parameterization=ee.enum.dcparam_option.torque_speed  Ra=r_motor Ohm  La=1 H  emf_or_torque=ee.enum.emf_or_torque.ki  Kv=YBT_Par.Pivot.Motor.K V/rpm  Ki=k_motor N*m/A  T_stall=0.0637 N*m  w_max=600 rpm  w_rated=1.5e+4 rpm  P_rated=0.08 W  V_rated=12 V  J=0 g*cm^2  lam_param=ee.enum.lam_param.current  lam=0 N*m/(rad/s)  i_noload=0.06 A  V_i_noload=12 V  speed0=0 rpm  alpha=3.93e-3 1/K  Tmeas=25 degC  thermal_mass=100 J/K  initial_temperature=25 degC
  Network : Subsystem
  PS-Simulink Converter : nesl_utility/PS-Simulink Converter  PhysicalDomain=network_engine_domain  SubClassName=ps_output  LeftPortType=input  RightPortType=output  PseudoPeriodic=off  Frequencies=[]  Unit=rad/s  AffineConversion=off
  Rotational Simscape Intf : Subsystem
  t : PMIOPort  Side=Left
  w : PMIOPort  Port=2  Side=Right
  - : PMIOPort  Port=3  Side=Right
  + : PMIOPort  Port=4  Side=Left
  wires:
  PS-Simulink Converter/1 -> Control/1(Meas)  "velocity"
  C/1 -> Control/2(Cmd)
  connections:
  Rotational Simscape Intf/RConn1 -- w/RConn1 -- PS-Simulink Converter/LConn1
  +/RConn1 -- Network/LConn2
  -/RConn1 -- Network/RConn1
  Motor/RConn1 -- Network/LConn1
  ERef H-Bridge/LConn1 -- H-Bridge/RConn2
  Control/RConn1 -- H-Bridge/LConn3
  Control/RConn2 -- Controlled Voltage/LConn1
  Motor/LConn1 -- H-Bridge/RConn1
  H-Bridge/LConn4 -- Controlled Voltage/LConn2 -- ERef/LConn1 -- H-Bridge/LConn2 -- Controlled Voltage/RConn2
  Controlled Voltage/RConn1 -- H-Bridge/LConn1
  t/RConn1 -- Rotational Simscape Intf/LConn1
  MRRef/LConn1 -- Rotational Simscape Intf/RConn2 -- Motor/RConn2
  Motor/LConn2 -- Gear/LConn1
  Rotational Simscape Intf/LConn2 -- Gear/RConn1

== system motor_model_final/DC MOTOR Speed Control/Motor1/Sensing i ==
  Current Sensor : fl_lib/Electrical/Electrical Sensors/Current Sensor
  i : PMIOPort  Side=Right
  + : PMIOPort  Port=2  Side=Left
  - : PMIOPort  Port=3  Side=Right
  connections:
  Current Sensor/LConn1 -- +/RConn1
  Current Sensor/RConn2 -- -/RConn1
  Current Sensor/RConn1 -- i/RConn1

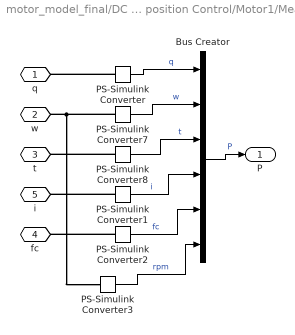
== system motor_model_final/DC MOTOR position Control/Motor1/Meas P ==
  Bus Creator : BusCreator  Inputs=6
  PS-Simulink Converter : nesl_utility/PS-Simulink Converter  PhysicalDomain=network_engine_domain  SubClassName=ps_output  LeftPortType=input  RightPortType=output  PseudoPeriodic=off  Frequencies=[]  Unit=rad  AffineConversion=off
  PS-Simulink Converter1 : nesl_utility/PS-Simulink Converter  PhysicalDomain=network_engine_domain  SubClassName=ps_output  LeftPortType=input  RightPortType=output  PseudoPeriodic=off  Frequencies=[]  Unit=A  AffineConversion=off
  PS-Simulink Converter2 : nesl_utility/PS-Simulink Converter  PhysicalDomain=network_engine_domain  SubClassName=ps_output  LeftPortType=input  RightPortType=output  PseudoPeriodic=off  Frequencies=[]  Unit=1  AffineConversion=off
  PS-Simulink Converter3 : nesl_utility/PS-Simulink Converter  PhysicalDomain=network_engine_domain  SubClassName=ps_output  LeftPortType=input  RightPortType=output  PseudoPeriodic=off  Frequencies=[]  Unit=rpm  AffineConversion=off
  PS-Simulink Converter7 : nesl_utility/PS-Simulink Converter  PhysicalDomain=network_engine_domain  SubClassName=ps_output  LeftPortType=input  RightPortType=output  PseudoPeriodic=off  Frequencies=[]  Unit=rad/s  AffineConversion=off
  PS-Simulink Converter8 : nesl_utility/PS-Simulink Converter  PhysicalDomain=network_engine_domain  SubClassName=ps_output  LeftPortType=input  RightPortType=output  PseudoPeriodic=off  Frequencies=[]  Unit=N*m  AffineConversion=off
  q : PMIOPort  Side=Left
  w : PMIOPort  Port=2  Side=Left
  t : PMIOPort  Port=3  Side=Left
  fc : PMIOPort  Port=4  Side=Left
  i : PMIOPort  Port=5  Side=Left
  P : Outport  VectorParamsAs1DForOutWhenUnconnected=off
  wires:
  Bus Creator/1 -> P/1  "P"
  PS-Simulink Converter8/1 -> Bus Creator/3  "t"
  PS-Simulink Converter7/1 -> Bus Creator/2  "w"
  PS-Simulink Converter/1 -> Bus Creator/1  "q"
  PS-Simulink Converter1/1 -> Bus Creator/4  "i"
  PS-Simulink Converter2/1 -> Bus Creator/5  "fc"
  PS-Simulink Converter3/1 -> Bus Creator/6  "rpm"
  connections:
  PS-Simulink Converter8/LConn1 -- t/RConn1
  PS-Simulink Converter/LConn1 -- q/RConn1
  PS-Simulink Converter1/LConn1 -- i/RConn1
  PS-Simulink Converter2/LConn1 -- fc/RConn1
  PS-Simulink Converter7/LConn1 -- PS-Simulink Converter3/LConn1 -- w/RConn1

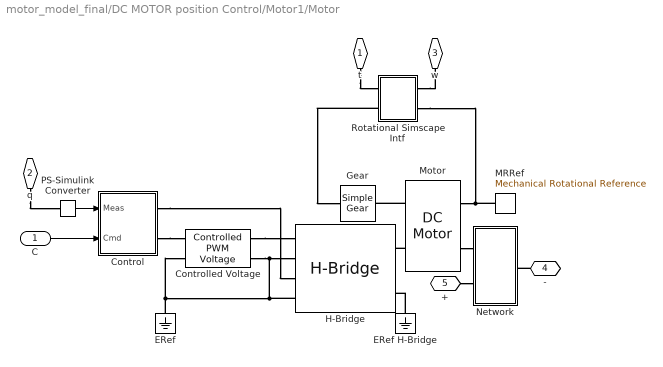
== system motor_model_final/DC MOTOR position Control/Motor1/Motor ==
  C : Inport  RequirementInfo={} %GIDa_368bb575_4ebf_43b9_b4ea_49c24a069202
  Control : Subsystem  RequirementInfo={} %GIDa_1ec0417b_7c76_4050_9d46_00f29d0701f9
  Controlled Voltage : ee_lib/Integrated Circuits/Controlled PWM Voltage  RequirementInfo={} %GIDa_73809545_7df6_434d_99db_e1e4c007496a  F=1000 Hz  TD=0 s  pulse_width_offset=0 s  pulse_min=0 s  Vmin=0 V  Vmax=5 V  Vm=5 V  pwm_or_av=2  event_type=1  sample_time=1e-6 s  u_min=0  u_max=1
  ERef : fl_lib/Electrical/Electrical Elements/Electrical Reference  RequirementInfo={} %GIDa_13c4472f_b89b_482f_9ffb_b40e92d1d3b6
  ERef H-Bridge : fl_lib/Electrical/Electrical Elements/Electrical Reference  RequirementInfo={} %GIDa_45275578_1c20_43d7_90b2_7bfacb70d4e2
  Gear : sdl_lib/Gears/Simple Gear  RequirementInfo={} %GIDa_08249044_1c97_412f_9f83_d43ac5b48ee2  ratio=1  rotation_direction=1  friction_model=sdl.enum.gear_efficiencies_load.off  T_noload=0.1 N*m  T_nom=5 N*m  efficiency_nom=0.8  efficiency=0.8  mu_visc=[ 0 0 ] N*m/(rad/s)  w_thr=0.01 rad/s  pwr_thr=0.001 W  enable_faults=simscape.enum.onoff.off  efficiency_fault=0.05  external_fault=simscape.enum.onoff.off  temporal_fault=simscape.enum.onoff.off  fault_time=5 s  fault_angles=pi / 12 rad  report_fault=1  temperature_TLU=[ 280 300 320 ] K  load_TLU=[ 1 5 10 ] N*m  efficiency_TLU=[ 0.95 0.9 0.85 ]  efficiency_TLU2=[ 0.85 0.8 0.75; 0.95 0.9 0.85; 0.85 0.8 0.7 ]  thermal_mass=50 J/K  T_init=300 K
  H-Bridge : ee_lib/Semiconductors & Converters/Converters/H-Bridge  RequirementInfo={} %GIDa_2d920dd3_d64f_4e64_9840_7eeb6e433ba1  supply_ports=ee.enum.supply_ports.hidesupply  Venable=2.5 V  Vmax=5.0 V  Vreverse=2.5 V  Vbrake=2.5 V  Vm=12 V  pwm_or_av=ee.enum.pwm_or_av.averaged  regenerative_braking_mode=ee.enum.converters.regenerative_braking_mode.always_enabled  discontinuous=ee.enum.current_profile.continuous  freewheeling_mode=ee.enum.converters.freewheeling_mode.one_switch_one_diode  Ron=0.1 Ohm  Don=0.05 Ohm  Goff=1e-6 S  Rload=10 Ohm  Lload=1e-5 H  F=10 kHz  thermal_mass=100 J/K  initial_temperature=298.15 K  Ron2=0.1 Ohm  Don2=0.05 Ohm  Tmeas=298.15 K  Tmeas2=398.15 K
  MRRef : fl_lib/Mechanical/Rotational Elements/Mechanical Rotational Reference  RequirementInfo={} %GIDa_f2f8a82a_ccb9_438c_b8d8_d7fb0f28210b
  Motor : ee_lib/Electromechanical/Brushed Motors/DC Motor  field_option=ee.enum.field_option.pm  Rf=100 Ohm  Lf=1 H  Laf=0.15 H  If0=0 A  parameterization=ee.enum.dcparam_option.torque_speed  Ra=r_motor Ohm  La=1 H  emf_or_torque=ee.enum.emf_or_torque.ki  Kv=YBT_Par.Pivot.Motor.K V/rpm  Ki=k_motor N*m/A  T_stall=0.0637 N*m  w_max=600 rpm  w_rated=1.5e+4 rpm  P_rated=0.08 W  V_rated=12 V  J=0 g*cm^2  lam_param=ee.enum.lam_param.current  lam=0 N*m/(rad/s)  i_noload=0.06 A  V_i_noload=12 V  speed0=0 rpm  alpha=3.93e-3 1/K  Tmeas=25 degC  thermal_mass=100 J/K  initial_temperature=25 degC
  Network : Subsystem  RequirementInfo={} %GIDa_9fee18e3_a948_413b_b883_e16fb674c0c0
  PS-Simulink Converter : nesl_utility/PS-Simulink Converter  RequirementInfo={} %GIDa_097674be_c2d9_46a2_88c8_91219fb03945  PhysicalDomain=network_engine_domain  SubClassName=ps_output  LeftPortType=input  RightPortType=output  PseudoPeriodic=off  Frequencies=[]  Unit=deg  AffineConversion=off
  Rotational Simscape Intf : Subsystem  RequirementInfo={} %GIDa_20a566a3_cdb1_4068_bc1b_4a204c2bcbb6
  t : PMIOPort  RequirementInfo={} %GIDa_a4b14222_3c31_477c_b014_3f812253a7d1  Side=Left
  q : PMIOPort  RequirementInfo={} %GIDa_573a934d_9532_4ee2_a8de_871da8711231  Port=2  Side=Right
  w : PMIOPort  RequirementInfo={} %GIDa_6a3eaa94_65d6_407b_b016_769070f6a746  Port=3  Side=Right
  - : PMIOPort  RequirementInfo={} %GIDa_ba051fe7_3f5b_4fff_b5df_531125b4f6cf  Port=4  Side=Right
  + : PMIOPort  RequirementInfo={} %GIDa_03fc6ed1_1d24_43d2_9ab2_d0402432e792  Port=5  Side=Left
  wires:
  C/1 -> Control/2(Cmd)
  PS-Simulink Converter/1 -> Control/1(Meas)
  connections:
  Rotational Simscape Intf/LConn2 -- Gear/RConn1
  Motor/LConn2 -- Gear/LConn1
  MRRef/LConn1 -- Motor/RConn2 -- Rotational Simscape Intf/RConn2
  t/RConn1 -- Rotational Simscape Intf/LConn1
  Controlled Voltage/RConn1 -- H-Bridge/LConn1
  Controlled Voltage/RConn2 -- H-Bridge/LConn2 -- ERef/LConn1 -- Controlled Voltage/LConn2 -- H-Bridge/LConn4
  Motor/LConn1 -- H-Bridge/RConn1
  Control/RConn2 -- Controlled Voltage/LConn1
  Control/RConn1 -- H-Bridge/LConn3
  ERef H-Bridge/LConn1 -- H-Bridge/RConn2
  Motor/RConn1 -- Network/LConn1
  -/RConn1 -- Network/RConn1
  +/RConn1 -- Network/LConn2
  q/RConn1 -- PS-Simulink Converter/LConn1
  Rotational Simscape Intf/RConn1 -- w/RConn1

== system motor_model_final/DC MOTOR position Control/Motor1/Sensing i ==
  Current Sensor : fl_lib/Electrical/Electrical Sensors/Current Sensor
  i : PMIOPort  Side=Right
  + : PMIOPort  Port=2  Side=Left
  - : PMIOPort  Port=3  Side=Right
  connections:
  Current Sensor/RConn1 -- i/RConn1
  Current Sensor/RConn2 -- -/RConn1
  Current Sensor/LConn1 -- +/RConn1

== system motor_model_final/DC MOTOR PWM Control/Motor1/Motor/Control ==
  PWM : Inport
  Abs : Abs  ZeroCross=off
  Gain : Gain  Gain=5/255
  Logic REV : Gain  Gain=5
  Saturation1 : Saturate  UpperLimit=255  LowerLimit=-255
  Sign : Signum  ZeroCross=off
  Voltage REV : Subsystem
  Voltage Ref : Subsystem
  REV : PMIOPort  Side=Right
  Ref : PMIOPort  Port=2  Side=Right
  wires:
  Gain/1 -> Sign/1, Abs/1
  Abs/1 -> Voltage Ref/1(SL)
  PWM/1 -> Saturation1/1
  Logic REV/1 -> Voltage REV/1(SL)
  Sign/1 -> Logic REV/1
  Saturation1/1 -> Gain/1
  connections:
  Voltage REV/RConn1 -- REV/RConn1
  Voltage Ref/RConn1 -- Ref/RConn1

== system motor_model_final/DC MOTOR PWM Control/Motor1/Motor/Network ==
  Abs : Abs  ZeroCross=off
  Current Sensor : fl_lib/Electrical/Electrical Sensors/Current Sensor
  Current Source : fl_lib/Electrical/Electrical Sources/Controlled Current Source
  ERef : fl_lib/Electrical/Electrical Elements/Electrical Reference
  PS-Simulink Converter : nesl_utility/PS-Simulink Converter  PhysicalDomain=network_engine_domain  SubClassName=ps_output  LeftPortType=input  RightPortType=output  PseudoPeriodic=off  Frequencies=[]  Unit=1  AffineConversion=off
  Simulink-PS Converter : nesl_utility/Simulink-PS Converter  PhysicalDomain=network_engine_domain  SubClassName=ps_input  LeftPortType=input  RightPortType=output  PseudoPeriodic=off  Frequencies=[]  NoiseDistribution=none  NoiseParameters=[]  Unit=1  AffineConversion=off  FilteringAndDerivatives=zero  SimscapeFilterOrder=1  InputFilterTimeConstant=0.005  UdotUserProvided=1
  " M" : PMIOPort  Side=Left
  - : PMIOPort  Port=2  Side=Right
  + : PMIOPort  Port=3  Side=Left
  wires:
  PS-Simulink Converter/1 -> Abs/1
  Abs/1 -> Simulink-PS Converter/1
  connections:
  -/RConn1 -- Current Source/LConn1
  +/RConn1 -- Current Source/RConn2
  Current Sensor/RConn1 -- PS-Simulink Converter/LConn1
  " M"/RConn1 -- Current Sensor/LConn1
  ERef/LConn1 -- Current Sensor/RConn2
  Simulink-PS Converter/RConn1 -- Current Source/RConn1

== system motor_model_final/DC MOTOR PWM Control/Motor1/Motor/Rotational Simscape Intf ==
  Angular Velocity Source : fl_lib/Mechanical/Mechanical Sources/Ideal Angular Velocity Source
  Torque Sensor : fl_lib/Mechanical/Mechanical Sensors/Ideal Torque Sensor
  w : PMIOPort  Side=Right
  t : PMIOPort  Port=2  Side=Left
  R : PMIOPort  Port=3  Side=Left
  C : PMIOPort  Port=4  Side=Right
  connections:
  w/RConn1 -- Angular Velocity Source/RConn1
  t/RConn1 -- Torque Sensor/RConn2
  Torque Sensor/LConn1 -- Angular Velocity Source/RConn2
  R/RConn1 -- Angular Velocity Source/LConn1
  Torque Sensor/RConn1 -- C/RConn1

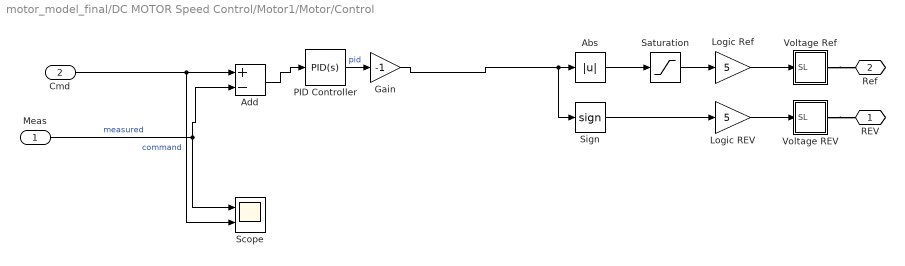
== system motor_model_final/DC MOTOR Speed Control/Motor1/Motor/Control ==
  Meas : Inport
  Cmd : Inport  Port=2
  Abs : Abs  ZeroCross=off
  Add : Sum  Inputs=+-
  Gain : Gain  Gain=-1
  Logic REV : Gain  Gain=5
  Logic Ref : Gain  Gain=5
  PID Controller : simulink/Continuous/PID Controller  Controller=PID  Form=Parallel  TimeDomain=Continuous-time  UseExternalTs=off  SampleTime=-1  IntegratorMethod=Forward Euler  FilterMethod=Forward Euler  ControllerParametersSource=internal  P=1.5  I=10  D=0.00001  UseFilter=on  N=100  TunerSelectOption=Transfer Function Based (PID Tuner App)  InitialConditionSource=internal  InitialConditionForIntegrator=0  InitialConditionForFilter=0  DifferentiatorICPrevScaledInput=0  ExternalReset=none  TrackingMode=off  Kt=1  LimitOutput=on  UpperSaturationLimit=1  LowerSaturationLimit=-1  LinearizeAsGain=on  AntiWindupMode=none  Kb=1  POutMin=[]  POutMax=[]  IOutMin=[]  IOutMax=[]  DOutMin=[]  DOutMax=[]  NOutMin=[]  NOutMax=[]  SumOutMin=[]  SumOutMax=[]  SaturationOutMin=[]  SaturationOutMax=[]  PParamMin=[]  PParamMax=[]  IParamMin=[]  IParamMax=[]  DParamMin=[]  DParamMax=[]  NParamMin=[]  NParamMax=[]  KbParamMin=[]  KbParamMax=[]  KtParamMin=[]  KtParamMax=[]  KbOutMin=[]  KbOutMax=[]  KtOutMin=[]  KtOutMax=[]  IntegratorOutMin=[]  IntegratorOutMax=[]  FilterOutMin=[]  FilterOutMax=[]  SumI1OutMin=[]  SumI1OutMax=[]  SumI2OutMin=[]  SumI2OutMax=[]  SumI3OutMin=[]  SumI3OutMax=[]  SumI4OutMin=[]  SumI4OutMax=[]  SumDOutMin=[]  SumDOutMax=[]  DifferentiatorOutMin=[]  DifferentiatorOutMax=[]  FilterDiffOutCoefMin=[]  FilterDiffOutCoefMax=[]  ReciprocalOutMin=[]  ReciprocalOutMax=[]  SumDenOutMin=[]  SumDenOutMax=[]  SumNumOutMin=[]  SumNumOutMax=[]  DivideOutMin=[]  DivideOutMax=[]  UdiffTsProdOutMin=[]  UdiffTsProdOutMax=[]  NTsProdOutMin=[]  NTsProdOutMax=[]  UintegralTsProdOutMin=[]  UintegralTsProdOutMax=[]  UngainTsProdOutMin=[]  UngainTsProdOutMax=[]  IntegratorContinuousStateAttributes=''  IntegratorStateMustResolveToSignalObject=off  IntegratorRTWStateStorageClass=Auto  FilterContinuousStateAttributes=''  FilterStateMustResolveToSignalObject=off  FilterRTWStateStorageClass=Auto  ParallelPVariant=InternalParameters  IdealPVariant=Disabled  IVariant=InternalParameters  DVariant=InternalParameters  IntegratorVariant=Continuous  SatVariant=Enabled  AWVariant=Passthrough  PCopyVariant=Disabled  TRVariant=Disabled  FdbkBlocksVariant=Forward  IdealPFdbkVariant=Disabled  SatFdbkVariant=Disabled  DerivativeFilterVariant=ContFilter  NVariant=InternalParameters  NCopyVariant=Disabled  FilterICVariant=InternalICsFilter  IntegratorICVariant=InternalICs  ExternalResetVariant=Disabled  TRSumVariant=Passthrough  SumFdbkVariant=Disabled  SumVariant=Sum_PID  TsampFilterVariant=InternalTs  TsampNgainVariant=Passthrough  TsampIntegralVariant=Passthrough
  Saturation : Saturate  UpperLimit=1  LowerLimit=0  ZeroCross=off
  Scope : Scope  NumInputPorts=2
  Sign : Signum  ZeroCross=off
  Voltage REV : Subsystem
  Voltage Ref : Subsystem
  REV : PMIOPort  Side=Right
  Ref : PMIOPort  Port=2  Side=Right
  wires:
  Logic Ref/1 -> Voltage Ref/1(SL)
  Logic REV/1 -> Voltage REV/1(SL)
  Sign/1 -> Logic REV/1
  Abs/1 -> Saturation/1
  Saturation/1 -> Logic Ref/1
  PID Controller/1 -> Gain/1  "pid"
  Add/1 -> PID Controller/1
  Meas/1 -> Scope/1, Add/2  "measured"
  Cmd/1 -> Scope/2, Add/1  "command"
  Gain/1 -> Sign/1, Abs/1
  connections:
  Voltage REV/RConn1 -- REV/RConn1
  Voltage Ref/RConn1 -- Ref/RConn1

== system motor_model_final/DC MOTOR Speed Control/Motor1/Motor/Network ==
  Abs : Abs  ZeroCross=off
  Current Sensor : fl_lib/Electrical/Electrical Sensors/Current Sensor
  Current Source : fl_lib/Electrical/Electrical Sources/Controlled Current Source
  ERef : fl_lib/Electrical/Electrical Elements/Electrical Reference
  PS-Simulink Converter : nesl_utility/PS-Simulink Converter  PhysicalDomain=network_engine_domain  SubClassName=ps_output  LeftPortType=input  RightPortType=output  PseudoPeriodic=off  Frequencies=[]  Unit=1  AffineConversion=off
  Simulink-PS Converter : nesl_utility/Simulink-PS Converter  PhysicalDomain=network_engine_domain  SubClassName=ps_input  LeftPortType=input  RightPortType=output  PseudoPeriodic=off  Frequencies=[]  NoiseDistribution=none  NoiseParameters=[]  Unit=1  AffineConversion=off  FilteringAndDerivatives=zero  SimscapeFilterOrder=1  InputFilterTimeConstant=0.005  UdotUserProvided=1
  " M" : PMIOPort  Side=Left
  - : PMIOPort  Port=2  Side=Right
  + : PMIOPort  Port=3  Side=Left
  wires:
  PS-Simulink Converter/1 -> Abs/1
  Abs/1 -> Simulink-PS Converter/1
  connections:
  -/RConn1 -- Current Source/LConn1
  +/RConn1 -- Current Source/RConn2
  Current Sensor/RConn1 -- PS-Simulink Converter/LConn1
  " M"/RConn1 -- Current Sensor/LConn1
  ERef/LConn1 -- Current Sensor/RConn2
  Simulink-PS Converter/RConn1 -- Current Source/RConn1

== system motor_model_final/DC MOTOR Speed Control/Motor1/Motor/Rotational Simscape Intf ==
  Angular Velocity Source : fl_lib/Mechanical/Mechanical Sources/Ideal Angular Velocity Source
  Torque Sensor : fl_lib/Mechanical/Mechanical Sensors/Ideal Torque Sensor
  w : PMIOPort  Side=Right
  t : PMIOPort  Port=2  Side=Left
  R : PMIOPort  Port=3  Side=Left
  C : PMIOPort  Port=4  Side=Right
  connections:
  w/RConn1 -- Angular Velocity Source/RConn1
  t/RConn1 -- Torque Sensor/RConn2
  Torque Sensor/LConn1 -- Angular Velocity Source/RConn2
  R/RConn1 -- Angular Velocity Source/LConn1
  Torque Sensor/RConn1 -- C/RConn1
